simulink library "xps_library"  (R2021a)
settings: Solver=VariableStepAuto  StartTime=0.0  StopTime=10.0  RelTol=1e-3
undefined symbols (not defined in the file or in its folder): ip_name, lib_path
libraries: xbsIndex_r4 x2612, casper_library_flow_control x68, simulink x52, $bdroot x9, casper_library_misc x9
(part 7 of 35)

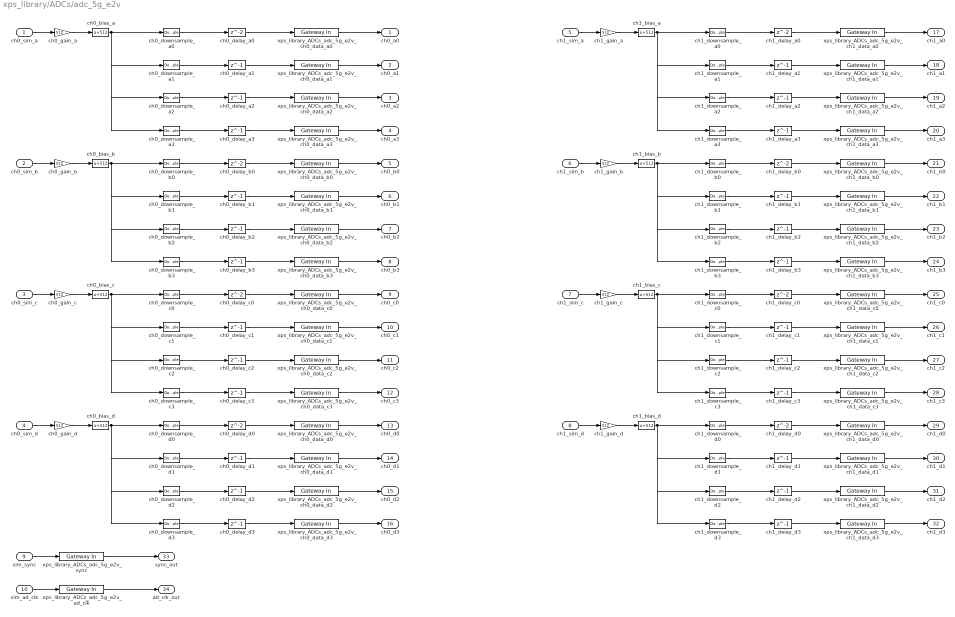
== system xps_library/ADCs/adc_5g_e2v ==
  ch0_sim_a : Inport
  ch0_sim_b : Inport  Port=2
  ch0_sim_c : Inport  Port=3
  ch0_sim_d : Inport  Port=4
  ch1_sim_a : Inport  Port=5
  ch1_sim_b : Inport  Port=6
  ch1_sim_c : Inport  Port=7
  ch1_sim_d : Inport  Port=8
  sim_sync : Inport  Port=9
  sim_ad_clk : Inport  Port=10
  ch0_bias_a : Bias  Bias=512  SaturateOnIntegerOverflow=on
  ch0_bias_b : Bias  Bias=512  SaturateOnIntegerOverflow=on
  ch0_bias_c : Bias  Bias=512  SaturateOnIntegerOverflow=on
  ch0_bias_d : Bias  Bias=512  SaturateOnIntegerOverflow=on
  ch0_delay_a0 : Delay  InitialCondition=0
  ch0_delay_a1 : Delay  DelayLength=1  InitialCondition=0
  ch0_delay_a2 : Delay  DelayLength=1  InitialCondition=0
  ch0_delay_a3 : Delay  DelayLength=1  InitialCondition=0
  ch0_delay_b0 : Delay  InitialCondition=0
  ch0_delay_b1 : Delay  DelayLength=1  InitialCondition=0
  ch0_delay_b2 : Delay  DelayLength=1  InitialCondition=0
  ch0_delay_b3 : Delay  DelayLength=1  InitialCondition=0
  ch0_delay_c0 : Delay  InitialCondition=0
  ch0_delay_c1 : Delay  DelayLength=1  InitialCondition=0
  ch0_delay_c2 : Delay  DelayLength=1  InitialCondition=0
  ch0_delay_c3 : Delay  DelayLength=1  InitialCondition=0
  ch0_delay_d0 : Delay  InitialCondition=0
  ch0_delay_d1 : Delay  DelayLength=1  InitialCondition=0
  ch0_delay_d2 : Delay  DelayLength=1  InitialCondition=0
  ch0_delay_d3 : Delay  DelayLength=1  InitialCondition=0
  ch0_downsample_a0 : DownSample  N=4  RateOptions=Allow multirate processing
  ch0_downsample_a1 : DownSample  N=4  phase=1  RateOptions=Allow multirate processing
  ch0_downsample_a2 : DownSample  N=4  phase=2  RateOptions=Allow multirate processing
  ch0_downsample_a3 : DownSample  N=4  phase=3  RateOptions=Allow multirate processing
  ch0_downsample_b0 : DownSample  N=4  RateOptions=Allow multirate processing
  ch0_downsample_b1 : DownSample  N=4  phase=1  RateOptions=Allow multirate processing
  ch0_downsample_b2 : DownSample  N=4  phase=2  RateOptions=Allow multirate processing
  ch0_downsample_b3 : DownSample  N=4  phase=3  RateOptions=Allow multirate processing
  ch0_downsample_c0 : DownSample  N=4  RateOptions=Allow multirate processing
  ch0_downsample_c1 : DownSample  N=4  phase=1  RateOptions=Allow multirate processing
  ch0_downsample_c2 : DownSample  N=4  phase=2  RateOptions=Allow multirate processing
  ch0_downsample_c3 : DownSample  N=4  phase=3  RateOptions=Allow multirate processing
  ch0_downsample_d0 : DownSample  N=4  RateOptions=Allow multirate processing
  ch0_downsample_d1 : DownSample  N=4  phase=1  RateOptions=Allow multirate processing
  ch0_downsample_d2 : DownSample  N=4  phase=2  RateOptions=Allow multirate processing
  ch0_downsample_d3 : DownSample  N=4  phase=3  RateOptions=Allow multirate processing
  ch0_gain_a : Gain  Gain=512  SaturateOnIntegerOverflow=on  OutDataTypeStr=Inherit: Same as input  ParamDataTypeStr=Inherit: Same as input
  ch0_gain_b : Gain  Gain=512  SaturateOnIntegerOverflow=on  OutDataTypeStr=Inherit: Same as input  ParamDataTypeStr=Inherit: Same as input
  ch0_gain_c : Gain  Gain=512  SaturateOnIntegerOverflow=on  OutDataTypeStr=Inherit: Same as input  ParamDataTypeStr=Inherit: Same as input
  ch0_gain_d : Gain  Gain=512  SaturateOnIntegerOverflow=on  OutDataTypeStr=Inherit: Same as input  ParamDataTypeStr=Inherit: Same as input
  ch1_bias_a : Bias  Bias=512  SaturateOnIntegerOverflow=on
  ch1_bias_b : Bias  Bias=512  SaturateOnIntegerOverflow=on
  ch1_bias_c : Bias  Bias=512  SaturateOnIntegerOverflow=on
  ch1_bias_d : Bias  Bias=512  SaturateOnIntegerOverflow=on
  ch1_delay_a0 : Delay  InitialCondition=0
  ch1_delay_a1 : Delay  DelayLength=1  InitialCondition=0
  ch1_delay_a2 : Delay  DelayLength=1  InitialCondition=0
  ch1_delay_a3 : Delay  DelayLength=1  InitialCondition=0
  ch1_delay_b0 : Delay  InitialCondition=0
  ch1_delay_b1 : Delay  DelayLength=1  InitialCondition=0
  ch1_delay_b2 : Delay  DelayLength=1  InitialCondition=0
  ch1_delay_b3 : Delay  DelayLength=1  InitialCondition=0
  ch1_delay_c0 : Delay  InitialCondition=0
  ch1_delay_c1 : Delay  DelayLength=1  InitialCondition=0
  ch1_delay_c2 : Delay  DelayLength=1  InitialCondition=0
  ch1_delay_c3 : Delay  DelayLength=1  InitialCondition=0
  ch1_delay_d0 : Delay  InitialCondition=0
  ch1_delay_d1 : Delay  DelayLength=1  InitialCondition=0
  ch1_delay_d2 : Delay  DelayLength=1  InitialCondition=0
  ch1_delay_d3 : Delay  DelayLength=1  InitialCondition=0
  ch1_downsample_a0 : DownSample  N=4  RateOptions=Allow multirate processing
  ch1_downsample_a1 : DownSample  N=4  phase=1  RateOptions=Allow multirate processing
  ch1_downsample_a2 : DownSample  N=4  phase=2  RateOptions=Allow multirate processing
  ch1_downsample_a3 : DownSample  N=4  phase=3  RateOptions=Allow multirate processing
  ch1_downsample_b0 : DownSample  N=4  RateOptions=Allow multirate processing
  ch1_downsample_b1 : DownSample  N=4  phase=1  RateOptions=Allow multirate processing
  ch1_downsample_b2 : DownSample  N=4  phase=2  RateOptions=Allow multirate processing
  ch1_downsample_b3 : DownSample  N=4  phase=3  RateOptions=Allow multirate processing
  ch1_downsample_c0 : DownSample  N=4  RateOptions=Allow multirate processing
  ch1_downsample_c1 : DownSample  N=4  phase=1  RateOptions=Allow multirate processing
  ch1_downsample_c2 : DownSample  N=4  phase=2  RateOptions=Allow multirate processing
  ch1_downsample_c3 : DownSample  N=4  phase=3  RateOptions=Allow multirate processing
  ch1_downsample_d0 : DownSample  N=4  RateOptions=Allow multirate processing
  ch1_downsample_d1 : DownSample  N=4  phase=1  RateOptions=Allow multirate processing
  ch1_downsample_d2 : DownSample  N=4  phase=2  RateOptions=Allow multirate processing
  ch1_downsample_d3 : DownSample  N=4  phase=3  RateOptions=Allow multirate processing
  ch1_gain_a : Gain  Gain=512  SaturateOnIntegerOverflow=on  OutDataTypeStr=Inherit: Same as input  ParamDataTypeStr=Inherit: Same as input
  ch1_gain_b : Gain  Gain=512  SaturateOnIntegerOverflow=on  OutDataTypeStr=Inherit: Same as input  ParamDataTypeStr=Inherit: Same as input
  ch1_gain_c : Gain  Gain=512  SaturateOnIntegerOverflow=on  OutDataTypeStr=Inherit: Same as input  ParamDataTypeStr=Inherit: Same as input
  ch1_gain_d : Gain  Gain=512  SaturateOnIntegerOverflow=on  OutDataTypeStr=Inherit: Same as input  ParamDataTypeStr=Inherit: Same as input
  xps_library_ADCs_adc_5g_e2v_ad_clk : xbsIndex_r4/Gateway In  gui_display_data_type=Fixed-point  arith_type=Boolean  n_bits=16  bin_pt=14  preci_type=Single  exp_width=8  frac_width=24  rows=1  columns=1  quantization="Round  (unbiased: +/- Inf)"  overflow=Saturate  period=1  UseAsADC=off  ADCChannel='1'  interface=None  automatic_assignment=on  address_offset=hex2dec('00')  intf_name=''  intf_description=''  default_value=0  timing_constraint=None  locs_specified=off  LOCs={}  io_standard={}  inherit_from_input=off  hdl_port=on  dbl_ovrd=off  block_type=gatewayin
  xps_library_ADCs_adc_5g_e2v_ch0_data_a{0..3} (4 alike) : xbsIndex_r4/Gateway In  gui_display_data_type=Fixed-point  arith_type=Unsigned  n_bits=10  bin_pt=0  preci_type=Single  exp_width=8  frac_width=24  rows=1  columns=1  quantization=Truncate  overflow=Wrap  period=1  UseAsADC=off  ADCChannel='1'  interface=None  automatic_assignment=on  address_offset=hex2dec('00')  intf_name=''  intf_description=''  default_value=0  timing_constraint=None  locs_specified=off  LOCs={}  io_standard={}  inherit_from_input=off  hdl_port=on  dbl_ovrd=off  block_type=gatewayin
  xps_library_ADCs_adc_5g_e2v_ch0_data_b{0..3} (4 alike) : xbsIndex_r4/Gateway In  gui_display_data_type=Fixed-point  arith_type=Unsigned  n_bits=10  bin_pt=0  preci_type=Single  exp_width=8  frac_width=24  rows=1  columns=1  quantization=Truncate  overflow=Wrap  period=1  UseAsADC=off  ADCChannel='1'  interface=None  automatic_assignment=on  address_offset=hex2dec('00')  intf_name=''  intf_description=''  default_value=0  timing_constraint=None  locs_specified=off  LOCs={}  io_standard={}  inherit_from_input=off  hdl_port=on  dbl_ovrd=off  block_type=gatewayin
  xps_library_ADCs_adc_5g_e2v_ch0_data_c{0..3} (4 alike) : xbsIndex_r4/Gateway In  gui_display_data_type=Fixed-point  arith_type=Unsigned  n_bits=10  bin_pt=0  preci_type=Single  exp_width=8  frac_width=24  rows=1  columns=1  quantization=Truncate  overflow=Wrap  period=1  UseAsADC=off  ADCChannel='1'  interface=None  automatic_assignment=on  address_offset=hex2dec('00')  intf_name=''  intf_description=''  default_value=0  timing_constraint=None  locs_specified=off  LOCs={}  io_standard={}  inherit_from_input=off  hdl_port=on  dbl_ovrd=off  block_type=gatewayin
  xps_library_ADCs_adc_5g_e2v_ch0_data_d{0..3} (4 alike) : xbsIndex_r4/Gateway In  gui_display_data_type=Fixed-point  arith_type=Unsigned  n_bits=10  bin_pt=0  preci_type=Single  exp_width=8  frac_width=24  rows=1  columns=1  quantization=Truncate  overflow=Wrap  period=1  UseAsADC=off  ADCChannel='1'  interface=None  automatic_assignment=on  address_offset=hex2dec('00')  intf_name=''  intf_description=''  default_value=0  timing_constraint=None  locs_specified=off  LOCs={}  io_standard={}  inherit_from_input=off  hdl_port=on  dbl_ovrd=off  block_type=gatewayin
  xps_library_ADCs_adc_5g_e2v_ch1_data_a{0..3} (4 alike) : xbsIndex_r4/Gateway In  gui_display_data_type=Fixed-point  arith_type=Unsigned  n_bits=10  bin_pt=0  preci_type=Single  exp_width=8  frac_width=24  rows=1  columns=1  quantization=Truncate  overflow=Wrap  period=1  UseAsADC=off  ADCChannel='1'  interface=None  automatic_assignment=on  address_offset=hex2dec('00')  intf_name=''  intf_description=''  default_value=0  timing_constraint=None  locs_specified=off  LOCs={}  io_standard={}  inherit_from_input=off  hdl_port=on  dbl_ovrd=off  block_type=gatewayin
  xps_library_ADCs_adc_5g_e2v_ch1_data_b{0..3} (4 alike) : xbsIndex_r4/Gateway In  gui_display_data_type=Fixed-point  arith_type=Unsigned  n_bits=10  bin_pt=0  preci_type=Single  exp_width=8  frac_width=24  rows=1  columns=1  quantization=Truncate  overflow=Wrap  period=1  UseAsADC=off  ADCChannel='1'  interface=None  automatic_assignment=on  address_offset=hex2dec('00')  intf_name=''  intf_description=''  default_value=0  timing_constraint=None  locs_specified=off  LOCs={}  io_standard={}  inherit_from_input=off  hdl_port=on  dbl_ovrd=off  block_type=gatewayin
  xps_library_ADCs_adc_5g_e2v_ch1_data_c{0..3} (4 alike) : xbsIndex_r4/Gateway In  gui_display_data_type=Fixed-point  arith_type=Unsigned  n_bits=10  bin_pt=0  preci_type=Single  exp_width=8  frac_width=24  rows=1  columns=1  quantization=Truncate  overflow=Wrap  period=1  UseAsADC=off  ADCChannel='1'  interface=None  automatic_assignment=on  address_offset=hex2dec('00')  intf_name=''  intf_description=''  default_value=0  timing_constraint=None  locs_specified=off  LOCs={}  io_standard={}  inherit_from_input=off  hdl_port=on  dbl_ovrd=off  block_type=gatewayin
  xps_library_ADCs_adc_5g_e2v_ch1_data_d{0..3} (4 alike) : xbsIndex_r4/Gateway In  gui_display_data_type=Fixed-point  arith_type=Unsigned  n_bits=10  bin_pt=0  preci_type=Single  exp_width=8  frac_width=24  rows=1  columns=1  quantization=Truncate  overflow=Wrap  period=1  UseAsADC=off  ADCChannel='1'  interface=None  automatic_assignment=on  address_offset=hex2dec('00')  intf_name=''  intf_description=''  default_value=0  timing_constraint=None  locs_specified=off  LOCs={}  io_standard={}  inherit_from_input=off  hdl_port=on  dbl_ovrd=off  block_type=gatewayin
  xps_library_ADCs_adc_5g_e2v_sync : xbsIndex_r4/Gateway In  gui_display_data_type=Fixed-point  arith_type=Boolean  n_bits=16  bin_pt=14  preci_type=Single  exp_width=8  frac_width=24  rows=1  columns=1  quantization="Round  (unbiased: +/- Inf)"  overflow=Saturate  period=1  UseAsADC=off  ADCChannel='1'  interface=None  automatic_assignment=on  address_offset=hex2dec('00')  intf_name=''  intf_description=''  default_value=0  timing_constraint=None  locs_specified=off  LOCs={}  io_standard={}  inherit_from_input=off  hdl_port=on  dbl_ovrd=off  block_type=gatewayin
  ch0_a0 : Outport  VectorParamsAs1DForOutWhenUnconnected=off
  ch0_a1 : Outport  Port=2  VectorParamsAs1DForOutWhenUnconnected=off
  ch0_a2 : Outport  Port=3  VectorParamsAs1DForOutWhenUnconnected=off
  ch0_a3 : Outport  Port=4  VectorParamsAs1DForOutWhenUnconnected=off
  ch0_b0 : Outport  Port=5  VectorParamsAs1DForOutWhenUnconnected=off
  ch0_b1 : Outport  Port=6  VectorParamsAs1DForOutWhenUnconnected=off
  ch0_b2 : Outport  Port=7  VectorParamsAs1DForOutWhenUnconnected=off
  ch0_b3 : Outport  Port=8  VectorParamsAs1DForOutWhenUnconnected=off
  ch0_c0 : Outport  Port=9  VectorParamsAs1DForOutWhenUnconnected=off
  ch0_c1 : Outport  Port=10  VectorParamsAs1DForOutWhenUnconnected=off
  ch0_c2 : Outport  Port=11  VectorParamsAs1DForOutWhenUnconnected=off
  ch0_c3 : Outport  Port=12  VectorParamsAs1DForOutWhenUnconnected=off
  ch0_d0 : Outport  Port=13  VectorParamsAs1DForOutWhenUnconnected=off
  ch0_d1 : Outport  Port=14  VectorParamsAs1DForOutWhenUnconnected=off
  ch0_d2 : Outport  Port=15  VectorParamsAs1DForOutWhenUnconnected=off
  ch0_d3 : Outport  Port=16  VectorParamsAs1DForOutWhenUnconnected=off
  ch1_a0 : Outport  Port=17  VectorParamsAs1DForOutWhenUnconnected=off
  ch1_a1 : Outport  Port=18  VectorParamsAs1DForOutWhenUnconnected=off
  ch1_a2 : Outport  Port=19  VectorParamsAs1DForOutWhenUnconnected=off
  ch1_a3 : Outport  Port=20  VectorParamsAs1DForOutWhenUnconnected=off
  ch1_b0 : Outport  Port=21  VectorParamsAs1DForOutWhenUnconnected=off
  ch1_b1 : Outport  Port=22  VectorParamsAs1DForOutWhenUnconnected=off
  ch1_b2 : Outport  Port=23  VectorParamsAs1DForOutWhenUnconnected=off
  ch1_b3 : Outport  Port=24  VectorParamsAs1DForOutWhenUnconnected=off
  ch1_c0 : Outport  Port=25  VectorParamsAs1DForOutWhenUnconnected=off
  ch1_c1 : Outport  Port=26  VectorParamsAs1DForOutWhenUnconnected=off
  ch1_c2 : Outport  Port=27  VectorParamsAs1DForOutWhenUnconnected=off
  ch1_c3 : Outport  Port=28  VectorParamsAs1DForOutWhenUnconnected=off
  ch1_d0 : Outport  Port=29  VectorParamsAs1DForOutWhenUnconnected=off
  ch1_d1 : Outport  Port=30  VectorParamsAs1DForOutWhenUnconnected=off
  ch1_d2 : Outport  Port=31  VectorParamsAs1DForOutWhenUnconnected=off
  ch1_d3 : Outport  Port=32  VectorParamsAs1DForOutWhenUnconnected=off
  sync_out : Outport  Port=33  VectorParamsAs1DForOutWhenUnconnected=off
  ad_clk_out : Outport  Port=34  VectorParamsAs1DForOutWhenUnconnected=off
  wires:
  ch0_sim_a/1 -> ch0_gain_a/1
  ch0_gain_a/1 -> ch0_bias_a/1
  ch0_bias_a/1 -> ch0_downsample_a0/1, ch0_downsample_a1/1, ch0_downsample_a2/1, ch0_downsample_a3/1
  ch0_downsample_a0/1 -> ch0_delay_a0/1
  ch0_delay_a0/1 -> xps_library_ADCs_adc_5g_e2v_ch0_data_a0/1
  xps_library_ADCs_adc_5g_e2v_ch0_data_a0/1 -> ch0_a0/1
  ch0_downsample_a1/1 -> ch0_delay_a1/1
  ch0_delay_a1/1 -> xps_library_ADCs_adc_5g_e2v_ch0_data_a1/1
  xps_library_ADCs_adc_5g_e2v_ch0_data_a1/1 -> ch0_a1/1
  ch0_downsample_a2/1 -> ch0_delay_a2/1
  ch0_delay_a2/1 -> xps_library_ADCs_adc_5g_e2v_ch0_data_a2/1
  xps_library_ADCs_adc_5g_e2v_ch0_data_a2/1 -> ch0_a2/1
  ch0_downsample_a3/1 -> ch0_delay_a3/1
  ch0_delay_a3/1 -> xps_library_ADCs_adc_5g_e2v_ch0_data_a3/1
  xps_library_ADCs_adc_5g_e2v_ch0_data_a3/1 -> ch0_a3/1
  ch0_sim_b/1 -> ch0_gain_b/1
  ch0_gain_b/1 -> ch0_bias_b/1
  ch0_bias_b/1 -> ch0_downsample_b0/1, ch0_downsample_b1/1, ch0_downsample_b2/1, ch0_downsample_b3/1
  ch0_downsample_b0/1 -> ch0_delay_b0/1
  ch0_delay_b0/1 -> xps_library_ADCs_adc_5g_e2v_ch0_data_b0/1
  xps_library_ADCs_adc_5g_e2v_ch0_data_b0/1 -> ch0_b0/1
  ch0_downsample_b1/1 -> ch0_delay_b1/1
  ch0_delay_b1/1 -> xps_library_ADCs_adc_5g_e2v_ch0_data_b1/1
  xps_library_ADCs_adc_5g_e2v_ch0_data_b1/1 -> ch0_b1/1
  ch0_downsample_b2/1 -> ch0_delay_b2/1
  ch0_delay_b2/1 -> xps_library_ADCs_adc_5g_e2v_ch0_data_b2/1
  xps_library_ADCs_adc_5g_e2v_ch0_data_b2/1 -> ch0_b2/1
  ch0_downsample_b3/1 -> ch0_delay_b3/1
  ch0_delay_b3/1 -> xps_library_ADCs_adc_5g_e2v_ch0_data_b3/1
  xps_library_ADCs_adc_5g_e2v_ch0_data_b3/1 -> ch0_b3/1
  ch0_sim_c/1 -> ch0_gain_c/1
  ch0_gain_c/1 -> ch0_bias_c/1
  ch0_bias_c/1 -> ch0_downsample_c0/1, ch0_downsample_c1/1, ch0_downsample_c2/1, ch0_downsample_c3/1
  ch0_downsample_c0/1 -> ch0_delay_c0/1
  ch0_delay_c0/1 -> xps_library_ADCs_adc_5g_e2v_ch0_data_c0/1
  xps_library_ADCs_adc_5g_e2v_ch0_data_c0/1 -> ch0_c0/1
  ch0_downsample_c1/1 -> ch0_delay_c1/1
  ch0_delay_c1/1 -> xps_library_ADCs_adc_5g_e2v_ch0_data_c1/1
  xps_library_ADCs_adc_5g_e2v_ch0_data_c1/1 -> ch0_c1/1
  ch0_downsample_c2/1 -> ch0_delay_c2/1
  ch0_delay_c2/1 -> xps_library_ADCs_adc_5g_e2v_ch0_data_c2/1
  xps_library_ADCs_adc_5g_e2v_ch0_data_c2/1 -> ch0_c2/1
  ch0_downsample_c3/1 -> ch0_delay_c3/1
  ch0_delay_c3/1 -> xps_library_ADCs_adc_5g_e2v_ch0_data_c3/1
  xps_library_ADCs_adc_5g_e2v_ch0_data_c3/1 -> ch0_c3/1
  ch0_sim_d/1 -> ch0_gain_d/1
  ch0_gain_d/1 -> ch0_bias_d/1
  ch0_bias_d/1 -> ch0_downsample_d0/1, ch0_downsample_d1/1, ch0_downsample_d2/1, ch0_downsample_d3/1
  ch0_downsample_d0/1 -> ch0_delay_d0/1
  ch0_delay_d0/1 -> xps_library_ADCs_adc_5g_e2v_ch0_data_d0/1
  xps_library_ADCs_adc_5g_e2v_ch0_data_d0/1 -> ch0_d0/1
  ch0_downsample_d1/1 -> ch0_delay_d1/1
  ch0_delay_d1/1 -> xps_library_ADCs_adc_5g_e2v_ch0_data_d1/1
  xps_library_ADCs_adc_5g_e2v_ch0_data_d1/1 -> ch0_d1/1
  ch0_downsample_d2/1 -> ch0_delay_d2/1
  ch0_delay_d2/1 -> xps_library_ADCs_adc_5g_e2v_ch0_data_d2/1
  xps_library_ADCs_adc_5g_e2v_ch0_data_d2/1 -> ch0_d2/1
  ch0_downsample_d3/1 -> ch0_delay_d3/1
  ch0_delay_d3/1 -> xps_library_ADCs_adc_5g_e2v_ch0_data_d3/1
  xps_library_ADCs_adc_5g_e2v_ch0_data_d3/1 -> ch0_d3/1
  ch1_sim_a/1 -> ch1_gain_a/1
  ch1_gain_a/1 -> ch1_bias_a/1
  ch1_bias_a/1 -> ch1_downsample_a0/1, ch1_downsample_a1/1, ch1_downsample_a2/1, ch1_downsample_a3/1
  ch1_downsample_a0/1 -> ch1_delay_a0/1
  ch1_delay_a0/1 -> xps_library_ADCs_adc_5g_e2v_ch1_data_a0/1
  xps_library_ADCs_adc_5g_e2v_ch1_data_a0/1 -> ch1_a0/1
  ch1_downsample_a1/1 -> ch1_delay_a1/1
  ch1_delay_a1/1 -> xps_library_ADCs_adc_5g_e2v_ch1_data_a1/1
  xps_library_ADCs_adc_5g_e2v_ch1_data_a1/1 -> ch1_a1/1
  ch1_downsample_a2/1 -> ch1_delay_a2/1
  ch1_delay_a2/1 -> xps_library_ADCs_adc_5g_e2v_ch1_data_a2/1
  xps_library_ADCs_adc_5g_e2v_ch1_data_a2/1 -> ch1_a2/1
  ch1_downsample_a3/1 -> ch1_delay_a3/1
  ch1_delay_a3/1 -> xps_library_ADCs_adc_5g_e2v_ch1_data_a3/1
  xps_library_ADCs_adc_5g_e2v_ch1_data_a3/1 -> ch1_a3/1
  ch1_sim_b/1 -> ch1_gain_b/1
  ch1_gain_b/1 -> ch1_bias_b/1
  ch1_bias_b/1 -> ch1_downsample_b0/1, ch1_downsample_b1/1, ch1_downsample_b2/1, ch1_downsample_b3/1
  ch1_downsample_b0/1 -> ch1_delay_b0/1
  ch1_delay_b0/1 -> xps_library_ADCs_adc_5g_e2v_ch1_data_b0/1
  xps_library_ADCs_adc_5g_e2v_ch1_data_b0/1 -> ch1_b0/1
  ch1_downsample_b1/1 -> ch1_delay_b1/1
  ch1_delay_b1/1 -> xps_library_ADCs_adc_5g_e2v_ch1_data_b1/1
  xps_library_ADCs_adc_5g_e2v_ch1_data_b1/1 -> ch1_b1/1
  ch1_downsample_b2/1 -> ch1_delay_b2/1
  ch1_delay_b2/1 -> xps_library_ADCs_adc_5g_e2v_ch1_data_b2/1
  xps_library_ADCs_adc_5g_e2v_ch1_data_b2/1 -> ch1_b2/1
  ch1_downsample_b3/1 -> ch1_delay_b3/1
  ch1_delay_b3/1 -> xps_library_ADCs_adc_5g_e2v_ch1_data_b3/1
  xps_library_ADCs_adc_5g_e2v_ch1_data_b3/1 -> ch1_b3/1
  ch1_sim_c/1 -> ch1_gain_c/1
  ch1_gain_c/1 -> ch1_bias_c/1
  ch1_bias_c/1 -> ch1_downsample_c0/1, ch1_downsample_c1/1, ch1_downsample_c2/1, ch1_downsample_c3/1
  ch1_downsample_c0/1 -> ch1_delay_c0/1
  ch1_delay_c0/1 -> xps_library_ADCs_adc_5g_e2v_ch1_data_c0/1
  xps_library_ADCs_adc_5g_e2v_ch1_data_c0/1 -> ch1_c0/1
  ch1_downsample_c1/1 -> ch1_delay_c1/1
  ch1_delay_c1/1 -> xps_library_ADCs_adc_5g_e2v_ch1_data_c1/1
  xps_library_ADCs_adc_5g_e2v_ch1_data_c1/1 -> ch1_c1/1
  ch1_downsample_c2/1 -> ch1_delay_c2/1
  ch1_delay_c2/1 -> xps_library_ADCs_adc_5g_e2v_ch1_data_c2/1
  xps_library_ADCs_adc_5g_e2v_ch1_data_c2/1 -> ch1_c2/1
  ch1_downsample_c3/1 -> ch1_delay_c3/1
  ch1_delay_c3/1 -> xps_library_ADCs_adc_5g_e2v_ch1_data_c3/1
  xps_library_ADCs_adc_5g_e2v_ch1_data_c3/1 -> ch1_c3/1
  ch1_sim_d/1 -> ch1_gain_d/1
  ch1_gain_d/1 -> ch1_bias_d/1
  ch1_bias_d/1 -> ch1_downsample_d0/1, ch1_downsample_d1/1, ch1_downsample_d2/1, ch1_downsample_d3/1
  ch1_downsample_d0/1 -> ch1_delay_d0/1
  ch1_delay_d0/1 -> xps_library_ADCs_adc_5g_e2v_ch1_data_d0/1
  xps_library_ADCs_adc_5g_e2v_ch1_data_d0/1 -> ch1_d0/1
  ch1_downsample_d1/1 -> ch1_delay_d1/1
  ch1_delay_d1/1 -> xps_library_ADCs_adc_5g_e2v_ch1_data_d1/1
  xps_library_ADCs_adc_5g_e2v_ch1_data_d1/1 -> ch1_d1/1
  ch1_downsample_d2/1 -> ch1_delay_d2/1
  ch1_delay_d2/1 -> xps_library_ADCs_adc_5g_e2v_ch1_data_d2/1
  xps_library_ADCs_adc_5g_e2v_ch1_data_d2/1 -> ch1_d2/1
  ch1_downsample_d3/1 -> ch1_delay_d3/1
  ch1_delay_d3/1 -> xps_library_ADCs_adc_5g_e2v_ch1_data_d3/1
  xps_library_ADCs_adc_5g_e2v_ch1_data_d3/1 -> ch1_d3/1
  sim_sync/1 -> xps_library_ADCs_adc_5g_e2v_sync/1
  xps_library_ADCs_adc_5g_e2v_sync/1 -> sync_out/1
  sim_ad_clk/1 -> xps_library_ADCs_adc_5g_e2v_ad_clk/1
  xps_library_ADCs_adc_5g_e2v_ad_clk/1 -> ad_clk_out/1

== system xps_library/ADCs/adc_mkid ==
  conv : Subsystem
      mask help:
      | Converts an (12-bit) unsigned number to 2's complement.
      | This block should eventually be able to handle arbitrary
      | width inputs.
  conv1 : Subsystem
      mask help:
      | Converts an (12-bit) unsigned number to 2's complement.
      | This block should eventually be able to handle arbitrary
      | width inputs.
  conv2 : Subsystem
      mask help:
      | Converts an (12-bit) unsigned number to 2's complement.
      | This block should eventually be able to handle arbitrary
      | width inputs.
  conv3 : Subsystem
      mask help:
      | Converts an (12-bit) unsigned number to 2's complement.
      | This block should eventually be able to handle arbitrary
      | width inputs.
  xps_library_ADCs_adc_mkid_user_data_i0 : xbsIndex_r4/Gateway In  gui_display_data_type=Fixed-point  arith_type=Unsigned  n_bits=12  bin_pt=0  preci_type=Single  exp_width=8  frac_width=24  rows=1  columns=1  quantization=Truncate  overflow=Wrap  period=1  UseAsADC=off  ADCChannel='1'  interface=None  automatic_assignment=on  address_offset=hex2dec('00')  intf_name=''  intf_description=''  default_value=0  timing_constraint=None  locs_specified=off  LOCs={}  io_standard={}  inherit_from_input=off  hdl_port=on  dbl_ovrd=off  block_type=gatewayin
      settings: infoedit="Gateway in block.  Converts inputs of type Simulink integer, double and fixed point to  Xilinx fixed point type.<P><P>Hardware notes:  In hardware these blocks become top level input ports."  xl_area=[0, 0, 0, 0, 0, 0, 0]  block_version=10.1.3
  xps_library_ADCs_adc_mkid_user_data_i1 : xbsIndex_r4/Gateway In  gui_display_data_type=Fixed-point  arith_type=Unsigned  n_bits=12  bin_pt=0  preci_type=Single  exp_width=8  frac_width=24  rows=1  columns=1  quantization=Truncate  overflow=Wrap  period=1  UseAsADC=off  ADCChannel='1'  interface=None  automatic_assignment=on  address_offset=hex2dec('00')  intf_name=''  intf_description=''  default_value=0  timing_constraint=None  locs_specified=off  LOCs={}  io_standard={}  inherit_from_input=off  hdl_port=on  dbl_ovrd=off  block_type=gatewayin
      settings: infoedit="Gateway in block.  Converts inputs of type Simulink integer, double and fixed point to  Xilinx fixed point type.<P><P>Hardware notes:  In hardware these blocks become top level input ports."  xl_area=[0, 0, 0, 0, 0, 0, 0]  block_version=10.1.3
  xps_library_ADCs_adc_mkid_user_data_q0 : xbsIndex_r4/Gateway In  gui_display_data_type=Fixed-point  arith_type=Unsigned  n_bits=12  bin_pt=0  preci_type=Single  exp_width=8  frac_width=24  rows=1  columns=1  quantization=Truncate  overflow=Wrap  period=1  UseAsADC=off  ADCChannel='1'  interface=None  automatic_assignment=on  address_offset=hex2dec('00')  intf_name=''  intf_description=''  default_value=0  timing_constraint=None  locs_specified=off  LOCs={}  io_standard={}  inherit_from_input=off  hdl_port=on  dbl_ovrd=off  block_type=gatewayin
      settings: infoedit="Gateway in block.  Converts inputs of type Simulink integer, double and fixed point to  Xilinx fixed point type.<P><P>Hardware notes:  In hardware these blocks become top level input ports."  xl_area=[0, 0, 0, 0, 0, 0, 0]  block_version=10.1.3
  xps_library_ADCs_adc_mkid_user_data_q1 : xbsIndex_r4/Gateway In  gui_display_data_type=Fixed-point  arith_type=Unsigned  n_bits=12  bin_pt=0  preci_type=Single  exp_width=8  frac_width=24  rows=1  columns=1  quantization=Truncate  overflow=Wrap  period=1  UseAsADC=off  ADCChannel='1'  interface=None  automatic_assignment=on  address_offset=hex2dec('00')  intf_name=''  intf_description=''  default_value=0  timing_constraint=None  locs_specified=off  LOCs={}  io_standard={}  inherit_from_input=off  hdl_port=on  dbl_ovrd=off  block_type=gatewayin
      settings: infoedit="Gateway in block.  Converts inputs of type Simulink integer, double and fixed point to  Xilinx fixed point type.<P><P>Hardware notes:  In hardware these blocks become top level input ports."  xl_area=[0, 0, 0, 0, 0, 0, 0]  block_version=10.1.3
  xps_library_ADCs_adc_mkid_user_sync : xbsIndex_r4/Gateway In  gui_display_data_type=Fixed-point  arith_type=Boolean  n_bits=1  bin_pt=0  preci_type=Single  exp_width=8  frac_width=24  rows=1  columns=1  quantization=Truncate  overflow=Wrap  period=1  UseAsADC=off  ADCChannel='1'  interface=None  automatic_assignment=on  address_offset=hex2dec('00')  intf_name=''  intf_description=''  default_value=0  timing_constraint=None  locs_specified=off  LOCs={}  io_standard={}  inherit_from_input=off  hdl_port=on  dbl_ovrd=off  block_type=gatewayin
      settings: infoedit="Gateway in block.  Converts inputs of type Simulink integer, double and fixed point to  Xilinx fixed point type.<P><P>Hardware notes:  In hardware these blocks become top level input ports."  xl_area=[0, 0, 0, 0, 0, 0, 0]  block_version=10.1.3
  data_i0 : Outport
  data_i1 : Outport  Port=2
  data_q0 : Outport  Port=3
  data_q1 : Outport  Port=4
  sync : Outport  Port=5
  wires:
  xps_library_ADCs_adc_mkid_user_sync/1 -> sync/1
  xps_library_ADCs_adc_mkid_user_data_i0/1 -> conv/1(In1)
  conv/1(Out1) -> data_i0/1
  xps_library_ADCs_adc_mkid_user_data_q0/1 -> conv2/1(In1)
  conv2/1(Out1) -> data_q0/1
  xps_library_ADCs_adc_mkid_user_data_i1/1 -> conv1/1(In1)
  conv1/1(Out1) -> data_i1/1
  xps_library_ADCs_adc_mkid_user_data_q1/1 -> conv3/1(In1)
  conv3/1(Out1) -> data_q1/1

== system xps_library/ADCs/adc_mkid_4x ==
  conv : Subsystem
      mask help:
      | Converts an (12-bit) unsigned number to 2's complement.
      | This block should eventually be able to handle arbitrary
      | width inputs.
  conv1 : Subsystem
      mask help:
      | Converts an (12-bit) unsigned number to 2's complement.
      | This block should eventually be able to handle arbitrary
      | width inputs.
  conv2 : Subsystem
      mask help:
      | Converts an (12-bit) unsigned number to 2's complement.
      | This block should eventually be able to handle arbitrary
      | width inputs.
  conv3 : Subsystem
      mask help:
      | Converts an (12-bit) unsigned number to 2's complement.
      | This block should eventually be able to handle arbitrary
      | width inputs.
  conv4 : Subsystem
      mask help:
      | Converts an (12-bit) unsigned number to 2's complement.
      | This block should eventually be able to handle arbitrary
      | width inputs.
  conv5 : Subsystem
      mask help:
      | Converts an (12-bit) unsigned number to 2's complement.
      | This block should eventually be able to handle arbitrary
      | width inputs.
  conv6 : Subsystem
      mask help:
      | Converts an (12-bit) unsigned number to 2's complement.
      | This block should eventually be able to handle arbitrary
      | width inputs.
  conv7 : Subsystem
      mask help:
      | Converts an (12-bit) unsigned number to 2's complement.
      | This block should eventually be able to handle arbitrary
      | width inputs.
  xps_library_ADCs_adc_mkid_4x_user_data_i{0..3} (4 alike) : xbsIndex_r4/Gateway In  gui_display_data_type=Fixed-point  arith_type=Unsigned  n_bits=12  bin_pt=0  preci_type=Single  exp_width=8  frac_width=24  rows=1  columns=1  quantization=Truncate  overflow=Wrap  period=1  UseAsADC=off  ADCChannel='1'  interface=None  automatic_assignment=on  address_offset=hex2dec('00')  intf_name=''  intf_description=''  default_value=0  timing_constraint=None  locs_specified=off  LOCs={}  io_standard={}  inherit_from_input=off  hdl_port=on  dbl_ovrd=off  block_type=gatewayin
      settings: infoedit="Gateway in block.  Converts inputs of type Simulink integer, double and fixed point to  Xilinx fixed point type.<P><P>Hardware notes:  In hardware these blocks become top level input ports."  xl_area=[0, 0, 0, 0, 0, 0, 0]  block_version=10.1.3
  xps_library_ADCs_adc_mkid_4x_user_data_q{0..3} (4 alike) : xbsIndex_r4/Gateway In  gui_display_data_type=Fixed-point  arith_type=Unsigned  n_bits=12  bin_pt=0  preci_type=Single  exp_width=8  frac_width=24  rows=1  columns=1  quantization=Truncate  overflow=Wrap  period=1  UseAsADC=off  ADCChannel='1'  interface=None  automatic_assignment=on  address_offset=hex2dec('00')  intf_name=''  intf_description=''  default_value=0  timing_constraint=None  locs_specified=off  LOCs={}  io_standard={}  inherit_from_input=off  hdl_port=on  dbl_ovrd=off  block_type=gatewayin
      settings: infoedit="Gateway in block.  Converts inputs of type Simulink integer, double and fixed point to  Xilinx fixed point type.<P><P>Hardware notes:  In hardware these blocks become top level input ports."  xl_area=[0, 0, 0, 0, 0, 0, 0]  block_version=10.1.3
  xps_library_ADCs_adc_mkid_4x_user_sync : xbsIndex_r4/Gateway In  gui_display_data_type=Fixed-point  arith_type=Boolean  n_bits=1  bin_pt=0  preci_type=Single  exp_width=8  frac_width=24  rows=1  columns=1  quantization=Truncate  overflow=Wrap  period=1  UseAsADC=off  ADCChannel='1'  interface=None  automatic_assignment=on  address_offset=hex2dec('00')  intf_name=''  intf_description=''  default_value=0  timing_constraint=None  locs_specified=off  LOCs={}  io_standard={}  inherit_from_input=off  hdl_port=on  dbl_ovrd=off  block_type=gatewayin
      settings: infoedit="Gateway in block.  Converts inputs of type Simulink integer, double and fixed point to  Xilinx fixed point type.<P><P>Hardware notes:  In hardware these blocks become top level input ports."  xl_area=[0, 0, 0, 0, 0, 0, 0]  block_version=10.1.3
  data_i0 : Outport
  data_i1 : Outport  Port=2
  data_i2 : Outport  Port=3
  data_i3 : Outport  Port=4
  data_q0 : Outport  Port=5
  data_q1 : Outport  Port=6
  data_q2 : Outport  Port=7
  data_q3 : Outport  Port=8
  sync : Outport  Port=9
  wires:
  xps_library_ADCs_adc_mkid_4x_user_data_q3/1 -> conv7/1(In1)
  conv7/1(Out1) -> data_q3/1
  xps_library_ADCs_adc_mkid_4x_user_data_q2/1 -> conv6/1(In1)
  conv6/1(Out1) -> data_q2/1
  xps_library_ADCs_adc_mkid_4x_user_data_i3/1 -> conv5/1(In1)
  conv5/1(Out1) -> data_i3/1
  xps_library_ADCs_adc_mkid_4x_user_data_i2/1 -> conv4/1(In1)
  conv4/1(Out1) -> data_i2/1
  xps_library_ADCs_adc_mkid_4x_user_sync/1 -> sync/1
  xps_library_ADCs_adc_mkid_4x_user_data_i0/1 -> conv/1(In1)
  conv/1(Out1) -> data_i0/1
  xps_library_ADCs_adc_mkid_4x_user_data_q0/1 -> conv2/1(In1)
  conv2/1(Out1) -> data_q0/1
  xps_library_ADCs_adc_mkid_4x_user_data_i1/1 -> conv1/1(In1)
  conv1/1(Out1) -> data_i1/1
  xps_library_ADCs_adc_mkid_4x_user_data_q1/1 -> conv3/1(In1)
  conv3/1(Out1) -> data_q1/1

== system xps_library/ADCs/adc_sim ==
  sim_adc_data_in : Inport
  adc_bias : Bias  Bias=128  SaturateOnIntegerOverflow=on
  adc_gain : Gain  Gain=128
  overflow_detector : $bdroot/ADCs/of_detect_bus  nStreams=8  bit_width=8
  sample0_ds : DownSample  N=8  phase=1
  sample1_ds : DownSample  N=8  phase=2
  sample2_ds : DownSample  N=8  phase=3
  sample3_ds : DownSample  N=8  phase=4
  sample4_ds : DownSample  N=8  phase=5
  sample5_ds : DownSample  N=8  phase=6
  sample6_ds : DownSample  N=8  phase=7
  sample7_ds : DownSample  N=8
  s0 : Outport
  s1 : Outport  Port=2
  s2 : Outport  Port=3
  s3 : Outport  Port=4
  s4 : Outport  Port=5
  s5 : Outport  Port=6
  s6 : Outport  Port=7
  s7 : Outport  Port=8
  of : Outport  Port=9
  wires:
  sim_adc_data_in/1 -> adc_gain/1
  adc_gain/1 -> adc_bias/1
  overflow_detector/1 -> of/1
  adc_bias/1 -> sample0_ds/1, sample1_ds/1, sample2_ds/1, sample3_ds/1, sample4_ds/1, sample5_ds/1, sample6_ds/1, sample7_ds/1
  sample0_ds/1 -> overflow_detector/1, s0/1
  sample1_ds/1 -> overflow_detector/2, s1/1
  sample2_ds/1 -> overflow_detector/3, s2/1
  sample3_ds/1 -> overflow_detector/4, s3/1
  sample4_ds/1 -> overflow_detector/5, s4/1
  sample5_ds/1 -> overflow_detector/6, s5/1
  sample6_ds/1 -> overflow_detector/7, s6/1
  sample7_ds/1 -> overflow_detector/8, s7/1

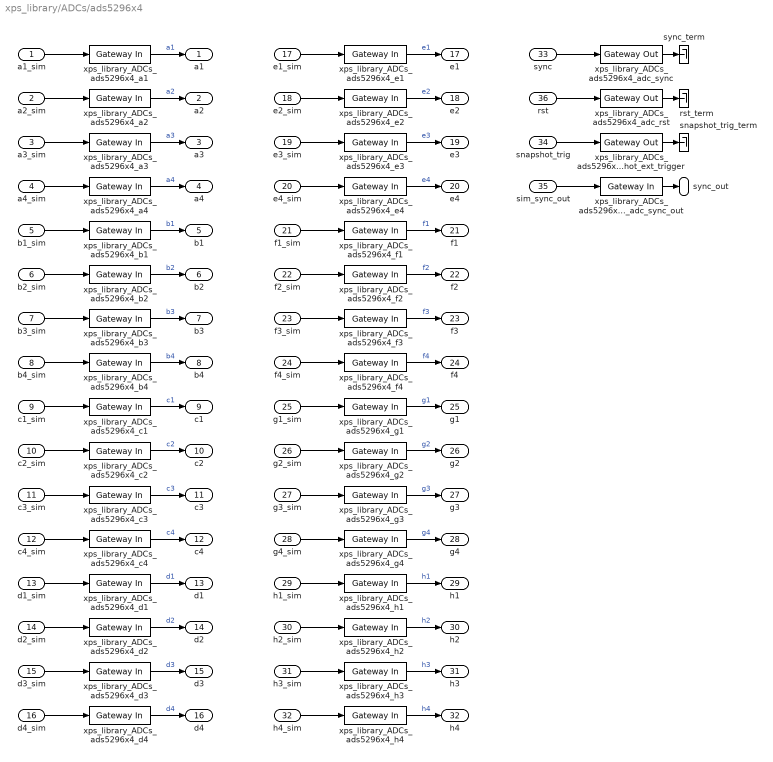
== system xps_library/ADCs/ads5296x4 ==
  a1_sim : Inport
  a2_sim : Inport  Port=2
  a3_sim : Inport  Port=3
  a4_sim : Inport  Port=4
  b1_sim : Inport  Port=5
  b2_sim : Inport  Port=6
  b3_sim : Inport  Port=7
  b4_sim : Inport  Port=8
  c1_sim : Inport  Port=9
  c2_sim : Inport  Port=10
  c3_sim : Inport  Port=11
  c4_sim : Inport  Port=12
  d1_sim : Inport  Port=13
  d2_sim : Inport  Port=14
  d3_sim : Inport  Port=15
  d4_sim : Inport  Port=16
  e1_sim : Inport  Port=17
  e2_sim : Inport  Port=18
  e3_sim : Inport  Port=19
  e4_sim : Inport  Port=20
  f1_sim : Inport  Port=21
  f2_sim : Inport  Port=22
  f3_sim : Inport  Port=23
  f4_sim : Inport  Port=24
  g1_sim : Inport  Port=25
  g2_sim : Inport  Port=26
  g3_sim : Inport  Port=27
  g4_sim : Inport  Port=28
  h1_sim : Inport  Port=29
  h2_sim : Inport  Port=30
  h3_sim : Inport  Port=31
  h4_sim : Inport  Port=32
  sync : Inport  Port=33
  snapshot_trig : Inport  Port=34
  sim_sync_out : Inport  Port=35
  rst : Inport  Port=36
  rst_term : Terminator
  snapshot_trig_term : Terminator
  sync_term : Terminator
  xps_library_ADCs_ads5296x4_a{1..4} (4 alike) : xbsIndex_r4/Gateway In  gui_display_data_type=Fixed-point  arith_type="Signed  (2's comp)"  n_bits=10  bin_pt=9  preci_type=Single  exp_width=8  frac_width=24  rows=1  columns=1  quantization="Round  (unbiased: +/- Inf)"  overflow=Saturate  period=1  UseAsADC=off  ADCChannel='1'  interface=None  automatic_assignment=on  address_offset=hex2dec('00')  intf_name=''  intf_description=''  default_value=0  timing_constraint=None  locs_specified=off  LOCs={}  io_standard={}  inherit_from_input=off  hdl_port=on  dbl_ovrd=off  block_type=gatewayin
  xps_library_ADCs_ads5296x4_adc_rst : xbsIndex_r4/Gateway Out  inherit_from_input=off  hdl_port=on  rows=1  columns=1  UseAsDAC=off  DACChannel='1'  interface=None  automatic_assignment=on  address_offset=hex2dec('00')  intf_name=''  intf_description=''  timing_constraint=None  locs_specified=off  LOCs={}  io_standard={}  block_type=gatewayout
  xps_library_ADCs_ads5296x4_adc_sync : xbsIndex_r4/Gateway Out  inherit_from_input=off  hdl_port=on  rows=1  columns=1  UseAsDAC=off  DACChannel='1'  interface=None  automatic_assignment=on  address_offset=hex2dec('00')  intf_name=''  intf_description=''  timing_constraint=None  locs_specified=off  LOCs={}  io_standard={}  block_type=gatewayout
  xps_library_ADCs_ads5296x4_adc_sync_out : xbsIndex_r4/Gateway In  gui_display_data_type=Fixed-point  arith_type=Boolean  n_bits=16  bin_pt=14  preci_type=Single  exp_width=8  frac_width=24  rows=1  columns=1  quantization="Round  (unbiased: +/- Inf)"  overflow=Saturate  period=1  UseAsADC=off  ADCChannel='1'  interface=None  automatic_assignment=on  address_offset=hex2dec('00')  intf_name=''  intf_description=''  default_value=0  timing_constraint=None  locs_specified=off  LOCs={}  io_standard={}  inherit_from_input=off  hdl_port=on  dbl_ovrd=off  block_type=gatewayin
  xps_library_ADCs_ads5296x4_b{1..4} (4 alike) : xbsIndex_r4/Gateway In  gui_display_data_type=Fixed-point  arith_type="Signed  (2's comp)"  n_bits=10  bin_pt=9  preci_type=Single  exp_width=8  frac_width=24  rows=1  columns=1  quantization="Round  (unbiased: +/- Inf)"  overflow=Saturate  period=1  UseAsADC=off  ADCChannel='1'  interface=None  automatic_assignment=on  address_offset=hex2dec('00')  intf_name=''  intf_description=''  default_value=0  timing_constraint=None  locs_specified=off  LOCs={}  io_standard={}  inherit_from_input=off  hdl_port=on  dbl_ovrd=off  block_type=gatewayin
  xps_library_ADCs_ads5296x4_c{1..4} (4 alike) : xbsIndex_r4/Gateway In  gui_display_data_type=Fixed-point  arith_type="Signed  (2's comp)"  n_bits=10  bin_pt=9  preci_type=Single  exp_width=8  frac_width=24  rows=1  columns=1  quantization="Round  (unbiased: +/- Inf)"  overflow=Saturate  period=1  UseAsADC=off  ADCChannel='1'  interface=None  automatic_assignment=on  address_offset=hex2dec('00')  intf_name=''  intf_description=''  default_value=0  timing_constraint=None  locs_specified=off  LOCs={}  io_standard={}  inherit_from_input=off  hdl_port=on  dbl_ovrd=off  block_type=gatewayin
  xps_library_ADCs_ads5296x4_d{1..4} (4 alike) : xbsIndex_r4/Gateway In  gui_display_data_type=Fixed-point  arith_type="Signed  (2's comp)"  n_bits=10  bin_pt=9  preci_type=Single  exp_width=8  frac_width=24  rows=1  columns=1  quantization="Round  (unbiased: +/- Inf)"  overflow=Saturate  period=1  UseAsADC=off  ADCChannel='1'  interface=None  automatic_assignment=on  address_offset=hex2dec('00')  intf_name=''  intf_description=''  default_value=0  timing_constraint=None  locs_specified=off  LOCs={}  io_standard={}  inherit_from_input=off  hdl_port=on  dbl_ovrd=off  block_type=gatewayin
  xps_library_ADCs_ads5296x4_e{1..4} (4 alike) : xbsIndex_r4/Gateway In  gui_display_data_type=Fixed-point  arith_type="Signed  (2's comp)"  n_bits=10  bin_pt=9  preci_type=Single  exp_width=8  frac_width=24  rows=1  columns=1  quantization="Round  (unbiased: +/- Inf)"  overflow=Saturate  period=1  UseAsADC=off  ADCChannel='1'  interface=None  automatic_assignment=on  address_offset=hex2dec('00')  intf_name=''  intf_description=''  default_value=0  timing_constraint=None  locs_specified=off  LOCs={}  io_standard={}  inherit_from_input=off  hdl_port=on  dbl_ovrd=off  block_type=gatewayin
  xps_library_ADCs_ads5296x4_f{1..4} (4 alike) : xbsIndex_r4/Gateway In  gui_display_data_type=Fixed-point  arith_type="Signed  (2's comp)"  n_bits=10  bin_pt=9  preci_type=Single  exp_width=8  frac_width=24  rows=1  columns=1  quantization="Round  (unbiased: +/- Inf)"  overflow=Saturate  period=1  UseAsADC=off  ADCChannel='1'  interface=None  automatic_assignment=on  address_offset=hex2dec('00')  intf_name=''  intf_description=''  default_value=0  timing_constraint=None  locs_specified=off  LOCs={}  io_standard={}  inherit_from_input=off  hdl_port=on  dbl_ovrd=off  block_type=gatewayin
  xps_library_ADCs_ads5296x4_g{1..4} (4 alike) : xbsIndex_r4/Gateway In  gui_display_data_type=Fixed-point  arith_type="Signed  (2's comp)"  n_bits=10  bin_pt=9  preci_type=Single  exp_width=8  frac_width=24  rows=1  columns=1  quantization="Round  (unbiased: +/- Inf)"  overflow=Saturate  period=1  UseAsADC=off  ADCChannel='1'  interface=None  automatic_assignment=on  address_offset=hex2dec('00')  intf_name=''  intf_description=''  default_value=0  timing_constraint=None  locs_specified=off  LOCs={}  io_standard={}  inherit_from_input=off  hdl_port=on  dbl_ovrd=off  block_type=gatewayin
  xps_library_ADCs_ads5296x4_h{1..4} (4 alike) : xbsIndex_r4/Gateway In  gui_display_data_type=Fixed-point  arith_type="Signed  (2's comp)"  n_bits=10  bin_pt=9  preci_type=Single  exp_width=8  frac_width=24  rows=1  columns=1  quantization="Round  (unbiased: +/- Inf)"  overflow=Saturate  period=1  UseAsADC=off  ADCChannel='1'  interface=None  automatic_assignment=on  address_offset=hex2dec('00')  intf_name=''  intf_description=''  default_value=0  timing_constraint=None  locs_specified=off  LOCs={}  io_standard={}  inherit_from_input=off  hdl_port=on  dbl_ovrd=off  block_type=gatewayin
  xps_library_ADCs_ads5296x4_snapshot_ext_trigger : xbsIndex_r4/Gateway Out  inherit_from_input=off  hdl_port=on  rows=1  columns=1  UseAsDAC=off  DACChannel='1'  interface=None  automatic_assignment=on  address_offset=hex2dec('00')  intf_name=''  intf_description=''  timing_constraint=None  locs_specified=off  LOCs={}  io_standard={}  block_type=gatewayout
  a1 : Outport  VectorParamsAs1DForOutWhenUnconnected=off
  a2 : Outport  Port=2  VectorParamsAs1DForOutWhenUnconnected=off
  a3 : Outport  Port=3  VectorParamsAs1DForOutWhenUnconnected=off
  a4 : Outport  Port=4  VectorParamsAs1DForOutWhenUnconnected=off
  b1 : Outport  Port=5  VectorParamsAs1DForOutWhenUnconnected=off
  b2 : Outport  Port=6  VectorParamsAs1DForOutWhenUnconnected=off
  b3 : Outport  Port=7  VectorParamsAs1DForOutWhenUnconnected=off
  b4 : Outport  Port=8  VectorParamsAs1DForOutWhenUnconnected=off
  c1 : Outport  Port=9  VectorParamsAs1DForOutWhenUnconnected=off
  c2 : Outport  Port=10  VectorParamsAs1DForOutWhenUnconnected=off
  c3 : Outport  Port=11  VectorParamsAs1DForOutWhenUnconnected=off
  c4 : Outport  Port=12  VectorParamsAs1DForOutWhenUnconnected=off
  d1 : Outport  Port=13  VectorParamsAs1DForOutWhenUnconnected=off
  d2 : Outport  Port=14  VectorParamsAs1DForOutWhenUnconnected=off
  d3 : Outport  Port=15  VectorParamsAs1DForOutWhenUnconnected=off
  d4 : Outport  Port=16  VectorParamsAs1DForOutWhenUnconnected=off
  e1 : Outport  Port=17  VectorParamsAs1DForOutWhenUnconnected=off
  e2 : Outport  Port=18  VectorParamsAs1DForOutWhenUnconnected=off
  e3 : Outport  Port=19  VectorParamsAs1DForOutWhenUnconnected=off
  e4 : Outport  Port=20  VectorParamsAs1DForOutWhenUnconnected=off
  f1 : Outport  Port=21  VectorParamsAs1DForOutWhenUnconnected=off
  f2 : Outport  Port=22  VectorParamsAs1DForOutWhenUnconnected=off
  f3 : Outport  Port=23  VectorParamsAs1DForOutWhenUnconnected=off
  f4 : Outport  Port=24  VectorParamsAs1DForOutWhenUnconnected=off
  g1 : Outport  Port=25  VectorParamsAs1DForOutWhenUnconnected=off
  g2 : Outport  Port=26  VectorParamsAs1DForOutWhenUnconnected=off
  g3 : Outport  Port=27  VectorParamsAs1DForOutWhenUnconnected=off
  g4 : Outport  Port=28  VectorParamsAs1DForOutWhenUnconnected=off
  h1 : Outport  Port=29  VectorParamsAs1DForOutWhenUnconnected=off
  h2 : Outport  Port=30  VectorParamsAs1DForOutWhenUnconnected=off
  h3 : Outport  Port=31  VectorParamsAs1DForOutWhenUnconnected=off
  h4 : Outport  Port=32  VectorParamsAs1DForOutWhenUnconnected=off
  sync_out : Outport  Port=33  VectorParamsAs1DForOutWhenUnconnected=off
  wires:
  a1_sim/1 -> xps_library_ADCs_ads5296x4_a1/1
  xps_library_ADCs_ads5296x4_a1/1 -> a1/1  "a1"
  a2_sim/1 -> xps_library_ADCs_ads5296x4_a2/1
  xps_library_ADCs_ads5296x4_a2/1 -> a2/1  "a2"
  a3_sim/1 -> xps_library_ADCs_ads5296x4_a3/1
  xps_library_ADCs_ads5296x4_a3/1 -> a3/1  "a3"
  a4_sim/1 -> xps_library_ADCs_ads5296x4_a4/1
  xps_library_ADCs_ads5296x4_a4/1 -> a4/1  "a4"
  b1_sim/1 -> xps_library_ADCs_ads5296x4_b1/1
  xps_library_ADCs_ads5296x4_b1/1 -> b1/1  "b1"
  b2_sim/1 -> xps_library_ADCs_ads5296x4_b2/1
  xps_library_ADCs_ads5296x4_b2/1 -> b2/1  "b2"
  b3_sim/1 -> xps_library_ADCs_ads5296x4_b3/1
  xps_library_ADCs_ads5296x4_b3/1 -> b3/1  "b3"
  b4_sim/1 -> xps_library_ADCs_ads5296x4_b4/1
  xps_library_ADCs_ads5296x4_b4/1 -> b4/1  "b4"
  c1_sim/1 -> xps_library_ADCs_ads5296x4_c1/1
  xps_library_ADCs_ads5296x4_c1/1 -> c1/1  "c1"
  c2_sim/1 -> xps_library_ADCs_ads5296x4_c2/1
  xps_library_ADCs_ads5296x4_c2/1 -> c2/1  "c2"
  c3_sim/1 -> xps_library_ADCs_ads5296x4_c3/1
  xps_library_ADCs_ads5296x4_c3/1 -> c3/1  "c3"
  c4_sim/1 -> xps_library_ADCs_ads5296x4_c4/1
  xps_library_ADCs_ads5296x4_c4/1 -> c4/1  "c4"
  d1_sim/1 -> xps_library_ADCs_ads5296x4_d1/1
  xps_library_ADCs_ads5296x4_d1/1 -> d1/1  "d1"
  d2_sim/1 -> xps_library_ADCs_ads5296x4_d2/1
  xps_library_ADCs_ads5296x4_d2/1 -> d2/1  "d2"
  d3_sim/1 -> xps_library_ADCs_ads5296x4_d3/1
  xps_library_ADCs_ads5296x4_d3/1 -> d3/1  "d3"
  d4_sim/1 -> xps_library_ADCs_ads5296x4_d4/1
  xps_library_ADCs_ads5296x4_d4/1 -> d4/1  "d4"
  e1_sim/1 -> xps_library_ADCs_ads5296x4_e1/1
  xps_library_ADCs_ads5296x4_e1/1 -> e1/1  "e1"
  e2_sim/1 -> xps_library_ADCs_ads5296x4_e2/1
  xps_library_ADCs_ads5296x4_e2/1 -> e2/1  "e2"
  e3_sim/1 -> xps_library_ADCs_ads5296x4_e3/1
  xps_library_ADCs_ads5296x4_e3/1 -> e3/1  "e3"
  e4_sim/1 -> xps_library_ADCs_ads5296x4_e4/1
  xps_library_ADCs_ads5296x4_e4/1 -> e4/1  "e4"
  f1_sim/1 -> xps_library_ADCs_ads5296x4_f1/1
  xps_library_ADCs_ads5296x4_f1/1 -> f1/1  "f1"
  f2_sim/1 -> xps_library_ADCs_ads5296x4_f2/1
  xps_library_ADCs_ads5296x4_f2/1 -> f2/1  "f2"
  f3_sim/1 -> xps_library_ADCs_ads5296x4_f3/1
  xps_library_ADCs_ads5296x4_f3/1 -> f3/1  "f3"
  f4_sim/1 -> xps_library_ADCs_ads5296x4_f4/1
  xps_library_ADCs_ads5296x4_f4/1 -> f4/1  "f4"
  g1_sim/1 -> xps_library_ADCs_ads5296x4_g1/1
  xps_library_ADCs_ads5296x4_g1/1 -> g1/1  "g1"
  g2_sim/1 -> xps_library_ADCs_ads5296x4_g2/1
  xps_library_ADCs_ads5296x4_g2/1 -> g2/1  "g2"
  g3_sim/1 -> xps_library_ADCs_ads5296x4_g3/1
  xps_library_ADCs_ads5296x4_g3/1 -> g3/1  "g3"
  g4_sim/1 -> xps_library_ADCs_ads5296x4_g4/1
  xps_library_ADCs_ads5296x4_g4/1 -> g4/1  "g4"
  h1_sim/1 -> xps_library_ADCs_ads5296x4_h1/1
  xps_library_ADCs_ads5296x4_h1/1 -> h1/1  "h1"
  h2_sim/1 -> xps_library_ADCs_ads5296x4_h2/1
  xps_library_ADCs_ads5296x4_h2/1 -> h2/1  "h2"
  h3_sim/1 -> xps_library_ADCs_ads5296x4_h3/1
  xps_library_ADCs_ads5296x4_h3/1 -> h3/1  "h3"
  h4_sim/1 -> xps_library_ADCs_ads5296x4_h4/1
  xps_library_ADCs_ads5296x4_h4/1 -> h4/1  "h4"
  sync/1 -> xps_library_ADCs_ads5296x4_adc_sync/1
  xps_library_ADCs_ads5296x4_adc_sync/1 -> sync_term/1
  rst/1 -> xps_library_ADCs_ads5296x4_adc_rst/1
  xps_library_ADCs_ads5296x4_adc_rst/1 -> rst_term/1
  snapshot_trig/1 -> xps_library_ADCs_ads5296x4_snapshot_ext_trigger/1
  xps_library_ADCs_ads5296x4_snapshot_ext_trigger/1 -> snapshot_trig_term/1
  sim_sync_out/1 -> xps_library_ADCs_ads5296x4_adc_sync_out/1
  xps_library_ADCs_ads5296x4_adc_sync_out/1 -> sync_out/1
